simulink model "Terminal_Voltage_Calculation"  (R2024a)
settings: Solver=VariableStepAuto  StartTime=0.0  StopTime=10.0  RelTol=1e-3
settings Model: Creator=ACER  LastModifiedBy=ACER

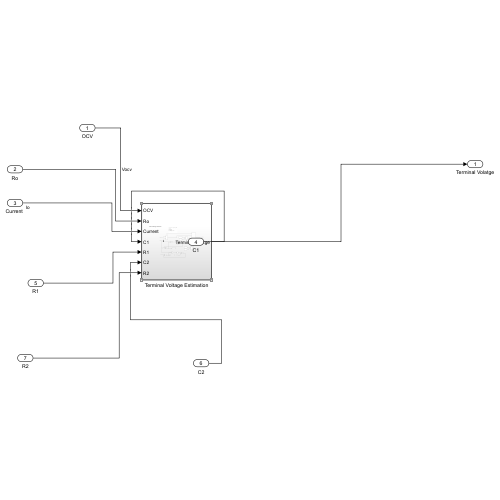
[thumbnail: Simulink's stored preview of the top-level diagram]
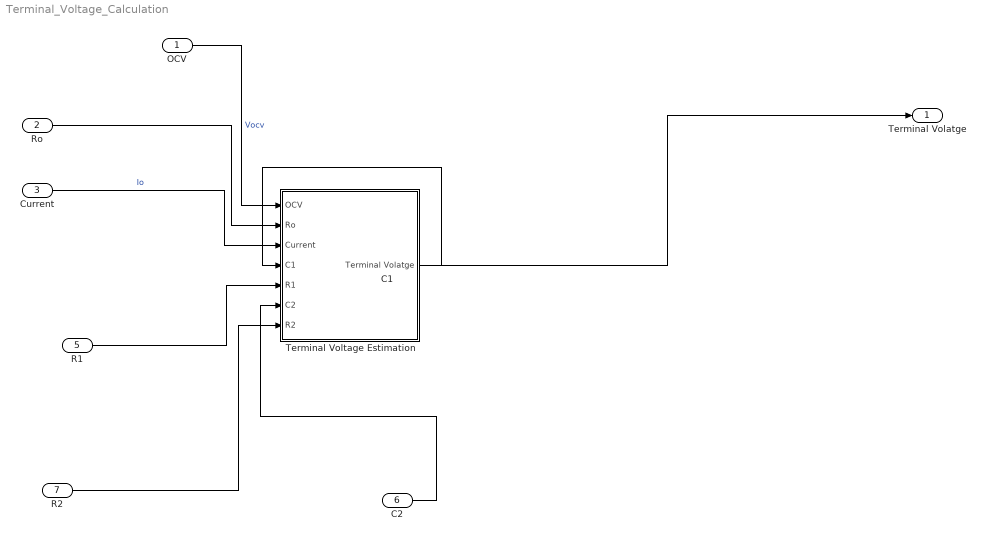
== system Terminal_Voltage_Calculation ==
  OCV : Inport
  Ro : Inport  Port=2
  "Current " : Inport  Port=3
  C1 : Inport  Port=4
  R1 : Inport  Port=5
  C2 : Inport  Port=6
  R2 : Inport  Port=7
  Terminal Voltage Estimation : Subsystem
  Terminal Volatge : Outport
  wires:
  OCV/1 -> Terminal Voltage Estimation/1(OCV)  "Vocv"
  Ro/1 -> Terminal Voltage Estimation/2(Ro)
  "Current "/1 -> Terminal Voltage Estimation/3("Current ")  "Io"
  C1/1 -> Terminal Voltage Estimation/4(C1)
  R1/1 -> Terminal Voltage Estimation/5(R1)
  C2/1 -> Terminal Voltage Estimation/6(C2)
  R2/1 -> Terminal Voltage Estimation/7(R2)
  Terminal Voltage Estimation/1(Terminal Volatge) -> Terminal Volatge/1

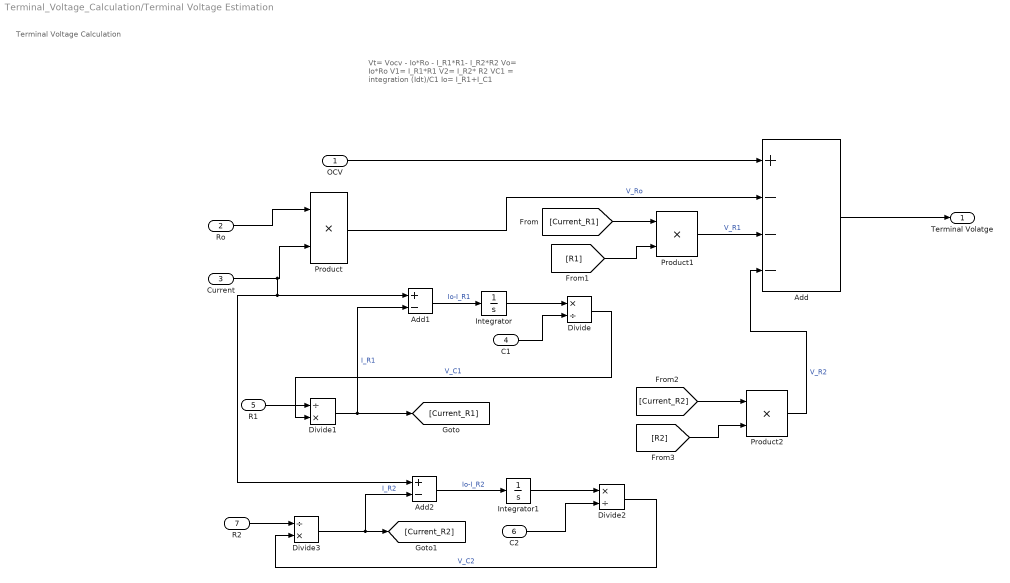
== system Terminal_Voltage_Calculation/Terminal Voltage Estimation ==
  note: Vt= Vocv - Io*Ro - I_R1*R1- I_R2*R2
      | Vo= Io*Ro
      | V1= I_R1*R1
      | V2= I_R2* R2
      | VC1 = integration (Idt)/C1
      | Io= I_R1+I_C1
  note: Terminal Voltage Calculation
  OCV : Inport
  Ro : Inport  Port=2
  "Current " : Inport  Port=3
  C1 : Inport  Port=4
  R1 : Inport  Port=5
  C2 : Inport  Port=6
  R2 : Inport  Port=7
  Add : Sum  Inputs=+---
  Add1 : Sum  Inputs=+-
  Add2 : Sum  Inputs=+-
  Divide : Product  Inputs=*/
  Divide1 : Product  Inputs=/*
  Divide2 : Product  Inputs=*/
  Divide3 : Product  Inputs=/*
  Integrator : Integrator
  Integrator1 : Integrator
  Product : Product
  Product1 : Product
  Product2 : Product
  Terminal Volatge : Outport
  wires:
  Add/1 -> Terminal Volatge/1
  Integrator/1 -> Divide/1
  Integrator1/1 -> Divide2/1
  R1/1 -> Divide1/1
  Add1/1 -> Integrator/1  "Io-I_R1"
  C1/1 -> Divide/2
  Ro/1 -> Product/1
  OCV/1 -> Add/1
  [Current_R2] -> Product2/1
  "Current "/1 -> Add2/1, Add1/1, Product/2
  [R2] -> Product2/2
  Add2/1 -> Integrator1/1  "Io-I_R2"
  R2/1 -> Divide3/1
  [Current_R1] -> Product1/1
  Product1/1 -> Add/3  "V_R1"
  Product/1 -> Add/2  "V_Ro"
  Divide3/1 -> [Current_R2], Add2/2  "I_R2"
  Divide2/1 -> Divide3/2  "V_C2"
  Divide1/1 -> [Current_R1], Add1/2  "I_R1"
  [R1] -> Product1/2
  Divide/1 -> Divide1/2  "V_C1"
  Product2/1 -> Add/4  "V_R2"
  C2/1 -> Divide2/2
